simulink model "Project_start_StateFlowFinal"  (R2023a)
settings: Solver=ode23t  StartTime=0.0  StopTime=300  RelTol=1e-3
InitFcn:
  | RPInit
model workspace (MAT data in the model file):
  mapForSim : object (value not decoded)
  occGrid : robotics.BinaryOccupancyGrid (value not decoded)
undefined symbols (not defined in the file): Base, FloorSurface, PlowSurface, Ref, RobotSurface, Side1, Side2, X, Y, Z
libraries: sm_lib x27, nesl_utility x11, RP_Simulator_Components x7, ME598_ProjectLibrary x3, RoboticsPlayground x2
(part 2 of 2)

== stateflow chart Project_start_StateFlowFinal/Chart ==
  state TurnLeft4
    L = -50;
    R = 50;
  state Forward9
    L = 50;
    R = 50;
  state TurnLeft5
    L = -50;
    R = 50;
  state Forward8
    L = 50;
    R = 50;
  state Reverse2
    L = -100;
    R = -100;
  state Turnleft
    L = -50;
    R = 50;
  state Forward7
    L = 50;
    R = 50;
  state TurnRight4
    L = 50;
    R = -50;
  state Forward
    L = 50;
    R = 50;
  state TurnRight
    L = 50;
    R = -50;
  state Forward1
    L = 50;
    R = 50;
  state TurnLeft2
    L = -50;
    R = 50;
  state Forward5
    L = 50
    R = 50
  state Reverse1
    L = -50
    R = -50
  state TurnLeft3
    L = -50
    R = 50
  state Forward6
    L = 50
    R = 50
  state TurnLeft
    L = -50;
    R = 50;
  state Forward3
    L = 50;
    R = 50;
  state TurnLeft1
    L = -50;
    R = 50;
  state Forward4
    L = 50;
    R = 50;
  state Reverse
    L = -50
    R = -50
  state TurnRight1
    L = 50
    R = -50
  state Reverse4
    L = -50
    R = -50
  state Forward13
    L = 50;
    R = 50;
  state TurnLeft7
    L = 50;
    R = -50;
  state Forward12
    L = 50;
    R = 50;
  state TurnLeft8
    L = 50;
    R =-50;
  state Stop1
    L=0;
    R=0;
  state Forward10
    L=50;
    R=50
  state TurnRight2
    L=50;
    R=-50;
  state Reverse3
    L=-50;
    R=-50;
  state Forward11
    L=50;
    R=50;
  state TurnRight3
    L=50;
    R=-50;
  state Stop
    L = 0
    R = 0
  state Forward15
    L = 50
    R = 50
  state TurnLeft9
    L = -50
    R = 50
  state Reverse5
    L = -50
    R = -50
  state Forward14
    L = 50
    R = 50
  state TurnLeft10
    L = -50;
    R = 50;
  state Forward16
    L = 50;
    R = 50;
  state TurnLeft11
    L = 50;
    R =-50;
  Forward9 -> TurnLeft5 : [X > 1.8]
  TurnLeft5 -> Forward8 : [theta > 90]
  TurnLeft4 -> Forward9 : [theta > -1 ]
  Reverse2 -> Turnleft : [Y < 0]
  Turnleft -> Forward7 : [theta > 177]
  Forward8 -> Reverse2 : [Forward < 0.7]
  Forward1 -> TurnLeft4 [order 3] : [RedDist < 0.4]
  Forward7 -> TurnRight4 : [X < 0]
  TurnRight4 -> Forward6 : [abs(theta) < 98]
  (default) -> Forward
  Forward -> TurnRight : [X > 0]
  TurnRight -> Forward1 : [theta < -87]
  Forward6 -> Stop : [BlueDist < 0.4 || GreenDist < 0.4 || RedDist < 0.4]
  Forward5 -> Reverse1 : [Forward < 0.7]
  TurnLeft2 -> Forward5 : [theta > -25]
  Reverse1 -> TurnLeft3 : [X < 0.05]
  Forward1 -> TurnLeft2 [order 2] : [GreenDist < 0.4]
  TurnLeft3 -> Forward6 : [theta > 85]
  Forward1 -> TurnLeft [order 1] : [BlueDist < 0.4]
  TurnRight1 -> Forward6 : [theta < 99]
  Forward4 -> Reverse : [Forward < 0.7]
  TurnLeft -> Forward3 : [theta > 88]
  TurnLeft1 -> Forward4 : [theta > 177]
  Forward3 -> TurnLeft1 : [Y >- 0.2 ]
  Reverse -> TurnRight1 : [X > -0.1]
  Reverse4 -> Stop1 : [X > 0]
  Forward12 -> TurnLeft7 : [Y <0.01 ]
  TurnLeft8 -> Forward12 : [theta < - 88]
  TurnLeft7 -> Forward13 : [theta  < -178]
  Stop -> TurnLeft8 [order 2] : [BlueDist < 0.4]
  Forward13 -> Reverse4 : [Forward < 0.7]
  Reverse3 -> TurnRight2 : [X < 0]
  TurnRight3 -> Forward11 : [theta < 25]
  Forward10 -> Stop1 : [Y < 0]
  TurnRight2 -> Forward10 : [theta < -85]
  Forward11 -> Reverse3 : [Forward < 0.7]
  Stop -> TurnRight3 [order 1] : [RedDist < 0.4]
  Forward15 -> Stop1 : [Y > 0]
  Stop -> TurnLeft11 [order 3] : [GreenDist < 0.4]
  Forward16 -> TurnLeft10 : [Y < -1.2]
  TurnLeft10 -> Forward14 : [theta > -25]
  Forward14 -> Reverse5 : [Forward < 0.7]
  Reverse5 -> TurnLeft9 : [X < 0.05]
  TurnLeft9 -> Forward15 : [theta > 85]
  TurnLeft11 -> Forward16 : [theta < - 88]
  data: theta input; L output; R output; BlueDist input; RedDist input; GreenDist input; Y input; X input; Forward input

== matlab function Project_start_StateFlowFinal/-180* : 180* ==
  data: deg input; deg output
function deg = degWrap(deg)

% % Convert radians to degrees
% deg = 180/pi * rad;


% Wrap degree value to the range -180* : +180*
for idx = 1:length(deg)
    while deg(idx) < -180
        deg(idx) = deg(idx)+360;
    end
    
    while deg(idx) > 180
        deg(idx) = deg(idx)-360;
    end
end

return
